simulink model "online_hardware_displacement_ctrl_arduino"  (R2020a)
settings: Solver=FixedStepAuto  StartTime=0.0  StopTime=25  FixedStep=0.01  RelTol=1e-3  EnableMultiTasking=on
libraries: simulink x4, arduinolib x4, arduinosensorlib x1
settings Model: SILPILModeSetting=veronly  ExtModeTrigDuration=2  Creator=Boreth  LastModifiedBy=Boreth
settings OptimizationCC: EnhancedBackFolding=on  PassReuseOutputArgsAs=Individual arguments  MaxStackSize=64  OptimizeBlockOrder=speed  DifferentSizesBufferReuse=on  EfficientTunableParamExpr=on
settings DebuggingCC: InheritedTsInSrcMsg=none  ParameterTunabilityLossMsg=error  ArithmeticOperatorsInVariantConditions=warning
settings HardwareCC: ProdBitPerPointer=32  ProdBitPerSizeT=32  ProdBitPerPtrDiffT=32  ProdLargestAtomicInteger=Long  ProdLargestAtomicFloat=Double  ProdWordSize=32  ProdHWDeviceType=ARM Compatible->ARM Cortex
settings SFSimCC: MATLABDynamicMemAlloc=off  CustomCodeUndefinedFunction=UseInterfaceOnly
settings RTWCC: SystemTargetFile=ert.tlc  HardwareBoard=Arduino Due  TLCOptions=-aInlineSetEventsForThisBaseRateFcn=TLC_FALSE -aSuppressMultiTaskScheduler=TLC_FALSE -aRateBasedStepFcn=1  TemplateMakefile=ert_default_tmf  GenerateReport=on  Toolchain=Arduino ARM  BuildConfiguration=Faster Runs  IncludeHyperlinkInReport=on  LaunchReport=on  GenerateTraceInfo=on  GenerateTraceReport=on  GenerateTraceReportSl=on  GenerateTraceReportSf=on  GenerateTraceReportEml=on
settings CodeAppCC: ForceParamTrailComments=on  IgnoreCustomStorageClasses=off  OperatorAnnotations=on  SimulinkDataObjDesc=on  SFDataObjDesc=on  InsertBlockDesc=on
settings ERTTargetCC: SupportContinuousTime=on  SupportVariableSizeSignals=on  ExtModeStaticAllocSize=24576

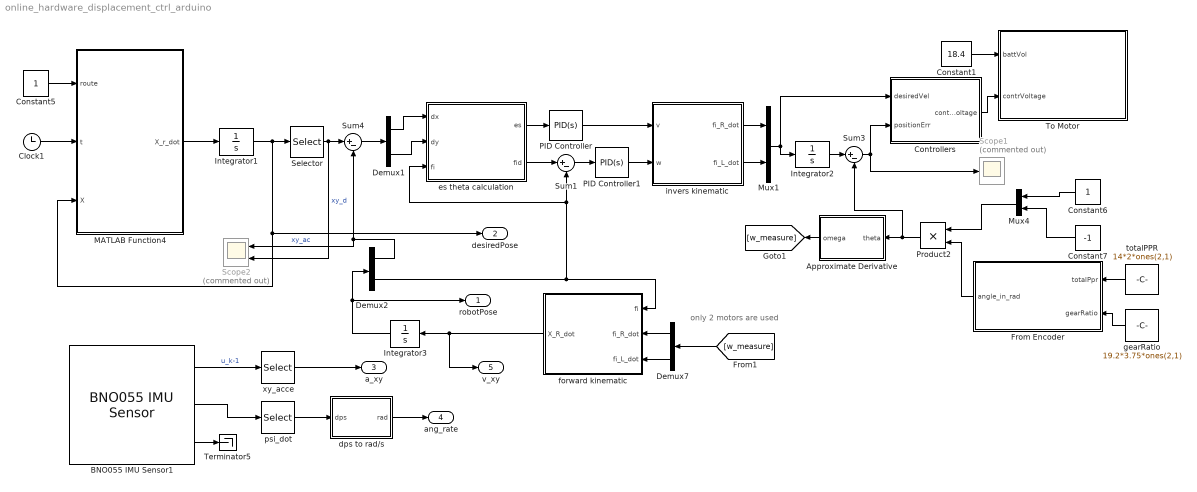
== system online_hardware_displacement_ctrl_arduino ==
  note: only 2 motors are used
  Approximate Derivative : Subsystem
  BNO055 IMU Sensor1 : arduinosensorlib/BNO055 IMU Sensor  SlaveAddress=0x28  OperationMode=Fusion  Accel=on  AngularRate=on  MagField=off  EulerAngles=off  Quat=off  LinearAccel=off  GravityVector=off  AccelRange=4G  AccelBW=62.5 Hz  GyroRange=2000 dps  GyroBW=32 Hz  MagODR=10 Hz  SampleTime=0.01  blockPlatform=ARDUINO
      settings: SourceProductName=Simulink Support Package for Arduino Hardware
  Clock1 : Clock
  Constant1 : Constant  Value=18.4
  Constant5 : Constant
  Constant6 : Constant
  Constant7 : Constant  Value=-1
  Controllers : Subsystem
  Demux1 : Demux  Outputs=2
  Demux2 : Demux  Outputs=[2 1]
  Demux7 : Demux  Outputs=2
  From Encoder : Subsystem
  Integrator1 : Integrator  InitialCondition=[0;0;0]
  Integrator2 : Integrator  InitialCondition=[0 0]
  Integrator3 : Integrator  InitialCondition=[0;0;0]
  MATLAB Function4 : MATLAB Function  TreatAsAtomicUnit=on
  Mux1 : Mux  Inputs=2
  Mux4 : Mux  Inputs=2
  PID Controller : simulink/Continuous/PID Controller  Controller=PID  Form=Parallel  TimeDomain=Continuous-time  UseExternalTs=off  SampleTime=-1  IntegratorMethod=Forward Euler  FilterMethod=Forward Euler  ControllerParametersSource=internal  P=0.35  I=0  D=0  UseFilter=on  N=100  TunerSelectOption=Transfer Function Based (PID Tuner App)  InitialConditionSource=internal  InitialConditionForIntegrator=0  InitialConditionForFilter=0  DifferentiatorICPrevScaledInput=0  ExternalReset=none  TrackingMode=off  Kt=1  LimitOutput=off  UpperSaturationLimit=inf  LowerSaturationLimit=-inf  LinearizeAsGain=on  AntiWindupMode=none  Kb=1  POutMin=[]  POutMax=[]  IOutMin=[]  IOutMax=[]  DOutMin=[]  DOutMax=[]  NOutMin=[]  NOutMax=[]  SumOutMin=[]  SumOutMax=[]  SaturationOutMin=[]  SaturationOutMax=[]  PParamMin=[]  PParamMax=[]  IParamMin=[]  IParamMax=[]  DParamMin=[]  DParamMax=[]  NParamMin=[]  NParamMax=[]  KbParamMin=[]  KbParamMax=[]  KtParamMin=[]  KtParamMax=[]  KbOutMin=[]  KbOutMax=[]  KtOutMin=[]  KtOutMax=[]  IntegratorOutMin=[]  IntegratorOutMax=[]  FilterOutMin=[]  FilterOutMax=[]  SumI1OutMin=[]  SumI1OutMax=[]  SumI2OutMin=[]  SumI2OutMax=[]  SumI3OutMin=[]  SumI3OutMax=[]  SumI4OutMin=[]  SumI4OutMax=[]  SumDOutMin=[]  SumDOutMax=[]  DifferentiatorOutMin=[]  DifferentiatorOutMax=[]  FilterDiffOutCoefMin=[]  FilterDiffOutCoefMax=[]  ReciprocalOutMin=[]  ReciprocalOutMax=[]  SumDenOutMin=[]  SumDenOutMax=[]  SumNumOutMin=[]  SumNumOutMax=[]  DivideOutMin=[]  DivideOutMax=[]  UdiffTsProdOutMin=[]  UdiffTsProdOutMax=[]  NTsProdOutMin=[]  NTsProdOutMax=[]  UintegralTsProdOutMin=[]  UintegralTsProdOutMax=[]  UngainTsProdOutMin=[]  UngainTsProdOutMax=[]  IntegratorContinuousStateAttributes=''  IntegratorStateMustResolveToSignalObject=off  IntegratorRTWStateStorageClass=Auto  FilterContinuousStateAttributes=''  FilterStateMustResolveToSignalObject=off  FilterRTWStateStorageClass=Auto  ParallelPVariant=InternalParameters  IdealPVariant=Disabled  IVariant=InternalParameters  DVariant=InternalParameters  IntegratorVariant=Continuous  SatVariant=Disabled  AWVariant=Passthrough  PCopyVariant=Disabled  TRVariant=Disabled  FdbkBlocksVariant=Forward  IdealPFdbkVariant=Disabled  SatFdbkVariant=Disabled  DerivativeFilterVariant=ContFilter  NVariant=InternalParameters  NCopyVariant=Disabled  FilterICVariant=InternalICsFilter  IntegratorICVariant=InternalICs  ExternalResetVariant=Disabled  TRSumVariant=Passthrough  SumFdbkVariant=Disabled  SumVariant=Sum_PID  TsampFilterVariant=InternalTs  TsampNgainVariant=Passthrough  TsampIntegralVariant=Passthrough
  PID Controller1 : simulink/Continuous/PID Controller  Controller=PID  Form=Parallel  TimeDomain=Continuous-time  UseExternalTs=off  SampleTime=-1  IntegratorMethod=Forward Euler  FilterMethod=Forward Euler  ControllerParametersSource=internal  P=3.2  I=0  D=0  UseFilter=on  N=100  TunerSelectOption=Transfer Function Based (PID Tuner App)  InitialConditionSource=internal  InitialConditionForIntegrator=0  InitialConditionForFilter=0  DifferentiatorICPrevScaledInput=0  ExternalReset=none  TrackingMode=off  Kt=1  LimitOutput=off  UpperSaturationLimit=inf  LowerSaturationLimit=-inf  LinearizeAsGain=on  AntiWindupMode=none  Kb=1  POutMin=[]  POutMax=[]  IOutMin=[]  IOutMax=[]  DOutMin=[]  DOutMax=[]  NOutMin=[]  NOutMax=[]  SumOutMin=[]  SumOutMax=[]  SaturationOutMin=[]  SaturationOutMax=[]  PParamMin=[]  PParamMax=[]  IParamMin=[]  IParamMax=[]  DParamMin=[]  DParamMax=[]  NParamMin=[]  NParamMax=[]  KbParamMin=[]  KbParamMax=[]  KtParamMin=[]  KtParamMax=[]  KbOutMin=[]  KbOutMax=[]  KtOutMin=[]  KtOutMax=[]  IntegratorOutMin=[]  IntegratorOutMax=[]  FilterOutMin=[]  FilterOutMax=[]  SumI1OutMin=[]  SumI1OutMax=[]  SumI2OutMin=[]  SumI2OutMax=[]  SumI3OutMin=[]  SumI3OutMax=[]  SumI4OutMin=[]  SumI4OutMax=[]  SumDOutMin=[]  SumDOutMax=[]  DifferentiatorOutMin=[]  DifferentiatorOutMax=[]  FilterDiffOutCoefMin=[]  FilterDiffOutCoefMax=[]  ReciprocalOutMin=[]  ReciprocalOutMax=[]  SumDenOutMin=[]  SumDenOutMax=[]  SumNumOutMin=[]  SumNumOutMax=[]  DivideOutMin=[]  DivideOutMax=[]  UdiffTsProdOutMin=[]  UdiffTsProdOutMax=[]  NTsProdOutMin=[]  NTsProdOutMax=[]  UintegralTsProdOutMin=[]  UintegralTsProdOutMax=[]  UngainTsProdOutMin=[]  UngainTsProdOutMax=[]  IntegratorContinuousStateAttributes=''  IntegratorStateMustResolveToSignalObject=off  IntegratorRTWStateStorageClass=Auto  FilterContinuousStateAttributes=''  FilterStateMustResolveToSignalObject=off  FilterRTWStateStorageClass=Auto  ParallelPVariant=InternalParameters  IdealPVariant=Disabled  IVariant=InternalParameters  DVariant=InternalParameters  IntegratorVariant=Continuous  SatVariant=Disabled  AWVariant=Passthrough  PCopyVariant=Disabled  TRVariant=Disabled  FdbkBlocksVariant=Forward  IdealPFdbkVariant=Disabled  SatFdbkVariant=Disabled  DerivativeFilterVariant=ContFilter  NVariant=InternalParameters  NCopyVariant=Disabled  FilterICVariant=InternalICsFilter  IntegratorICVariant=InternalICs  ExternalResetVariant=Disabled  TRSumVariant=Passthrough  SumFdbkVariant=Disabled  SumVariant=Sum_PID  TsampFilterVariant=InternalTs  TsampNgainVariant=Passthrough  TsampIntegralVariant=Passthrough
  Product2 : Product
  Scope1 : Scope  Commented=on
  Scope2 : Scope  Commented=on  NumInputPorts=2
  Selector : Selector  InputPortWidth=3  IndexOptions=Index vector (dialog)  Indices=[1 2]  OutputSizes=1
  Sum1 : Sum  Inputs=|+-
  Sum3 : Sum  Inputs=|+-
  Sum4 : Sum  Inputs=|+-
  Terminator5 : Terminator
  To Motor : Subsystem
  dps to rad/s : MATLAB Function  TreatAsAtomicUnit=on
  es theta calculation : MATLAB Function  TreatAsAtomicUnit=on
  forward kinematic : MATLAB Function  TreatAsAtomicUnit=on
  gearRatio : Constant  Value=19.2*3.75*ones(2,1)
  invers kinematic : MATLAB Function  TreatAsAtomicUnit=on
  psi_dot : Selector  InputPortWidth=3  IndexOptions=Index vector (dialog)  Indices=3  OutputSizes=1
  totalPPR : Constant  Value=14*2*ones(2,1)
  xy_acce : Selector  InputPortWidth=3  IndexOptions=Index vector (dialog)  Indices=[1 2]  OutputSizes=1
  robotPose : Outport
  desiredPose : Outport  Port=2
  a_xy : Outport  Port=3
  ang_rate : Outport  Port=4
  v_xy : Outport  Port=5
  wires:
  Approximate Derivative/1(omega) -> [w_measure]
  Controllers/1(contrVoltage) -> To Motor/2(contrVoltage)
  Mux1/1 -> Controllers/1(desiredVel), Integrator2/1
  Integrator2/1 -> Sum3/1
  From Encoder/1(angle_in_rad) -> Product2/2
  Sum3/1 -> Scope1/1, Controllers/2(positionErr)
  Mux4/1 -> Product2/1
  Product2/1 -> Sum3/2, Approximate Derivative/1(theta)
  Constant7/1 -> Mux4/2
  Constant6/1 -> Mux4/1
  BNO055 IMU Sensor1/3 -> Terminator5/1
  xy_acce/1 -> a_xy/1
  dps to rad/s/1(rad) -> ang_rate/1
  BNO055 IMU Sensor1/1 -> xy_acce/1  "u_k-1"
  psi_dot/1 -> dps to rad/s/1(dps)
  BNO055 IMU Sensor1/2 -> psi_dot/1
  forward kinematic/1(X_R_dot) -> v_xy/1, Integrator3/1
  Selector/1 -> Scope2/2, Sum4/1  "xy_d"
  PID Controller1/1 -> invers kinematic/2(w)
  Demux1/1 -> es theta calculation/1(dx)
  Demux1/2 -> es theta calculation/2(dy)
  MATLAB Function4/1(X_r_dot) -> Integrator1/1
  es theta calculation/2(fid) -> Sum1/1
  PID Controller/1 -> invers kinematic/1(v)
  Sum4/1 -> Demux1/1
  Demux2/2 -> es theta calculation/3(fi), Sum1/2, forward kinematic/1(fi)
  Sum1/1 -> PID Controller1/1
  es theta calculation/1(es) -> PID Controller/1
  Demux7/1 -> forward kinematic/2(fi_R_dot)
  Demux2/1 -> Scope2/1, Sum4/2  "xy_ac"
  invers kinematic/1(fi_R_dot) -> Mux1/1
  Demux7/2 -> forward kinematic/3(fi_L_dot)
  Integrator3/1 -> Demux2/1, robotPose/1
  invers kinematic/2(fi_L_dot) -> Mux1/2
  Clock1/1 -> MATLAB Function4/2(t)
  Integrator1/1 -> Selector/1, desiredPose/1, MATLAB Function4/3(X)
  Constant5/1 -> MATLAB Function4/1(route)
  [w_measure] -> Demux7/1
  totalPPR/1 -> From Encoder/1(totalPpr)
  gearRatio/1 -> From Encoder/2(gearRatio)
  Constant1/1 -> To Motor/1(battVol)

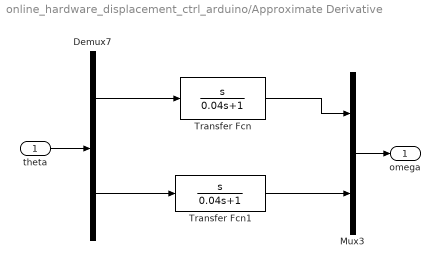
== system online_hardware_displacement_ctrl_arduino/Approximate Derivative ==
  theta : Inport
  Demux7 : Demux  Outputs=2
  Mux3 : Mux  Inputs=2
  Transfer Fcn : TransferFcn  Numerator=[1 0]  Denominator=[0.04 1]
  Transfer Fcn1 : TransferFcn  Numerator=[1 0]  Denominator=[0.04 1]
  omega : Outport
  wires:
  Transfer Fcn1/1 -> Mux3/2
  Transfer Fcn/1 -> Mux3/1
  Mux3/1 -> omega/1
  Demux7/1 -> Transfer Fcn/1
  Demux7/2 -> Transfer Fcn1/1
  theta/1 -> Demux7/1

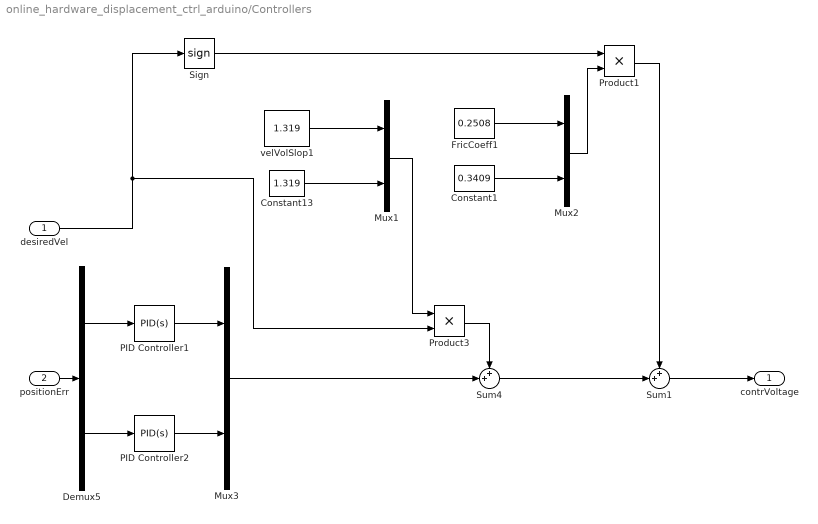
== system online_hardware_displacement_ctrl_arduino/Controllers ==
  desiredVel : Inport
  positionErr : Inport  Port=2
  Constant1 : Constant  Value=0.3409
  Constant13 : Constant  Value=1.319
  Demux5 : Demux  Outputs=2
  FricCoeff1 : Constant  Value=0.2508
  Mux1 : Mux  Inputs=2
  Mux2 : Mux  Inputs=2
  Mux3 : Mux  Inputs=2
  "PID Controller1 " : simulink/Continuous/PID Controller  Controller=PID  Form=Parallel  TimeDomain=Continuous-time  UseExternalTs=off  SampleTime=-1  IntegratorMethod=Forward Euler  FilterMethod=Forward Euler  ControllerParametersSource=internal  P=60  I=0  D=3  UseFilter=on  N=50  TunerSelectOption=Transfer Function Based (PID Tuner App)  InitialConditionSource=internal  InitialConditionForIntegrator=0  InitialConditionForFilter=0  DifferentiatorICPrevScaledInput=0  ExternalReset=none  TrackingMode=off  Kt=1  LimitOutput=off  UpperSaturationLimit=inf  LowerSaturationLimit=-inf  LinearizeAsGain=on  AntiWindupMode=none  Kb=1  POutMin=[]  POutMax=[]  IOutMin=[]  IOutMax=[]  DOutMin=[]  DOutMax=[]  NOutMin=[]  NOutMax=[]  SumOutMin=[]  SumOutMax=[]  SaturationOutMin=[]  SaturationOutMax=[]  PParamMin=[]  PParamMax=[]  IParamMin=[]  IParamMax=[]  DParamMin=[]  DParamMax=[]  NParamMin=[]  NParamMax=[]  KbParamMin=[]  KbParamMax=[]  KtParamMin=[]  KtParamMax=[]  KbOutMin=[]  KbOutMax=[]  KtOutMin=[]  KtOutMax=[]  IntegratorOutMin=[]  IntegratorOutMax=[]  FilterOutMin=[]  FilterOutMax=[]  SumI1OutMin=[]  SumI1OutMax=[]  SumI2OutMin=[]  SumI2OutMax=[]  SumI3OutMin=[]  SumI3OutMax=[]  SumI4OutMin=[]  SumI4OutMax=[]  SumDOutMin=[]  SumDOutMax=[]  DifferentiatorOutMin=[]  DifferentiatorOutMax=[]  FilterDiffOutCoefMin=[]  FilterDiffOutCoefMax=[]  ReciprocalOutMin=[]  ReciprocalOutMax=[]  SumDenOutMin=[]  SumDenOutMax=[]  SumNumOutMin=[]  SumNumOutMax=[]  DivideOutMin=[]  DivideOutMax=[]  UdiffTsProdOutMin=[]  UdiffTsProdOutMax=[]  NTsProdOutMin=[]  NTsProdOutMax=[]  UintegralTsProdOutMin=[]  UintegralTsProdOutMax=[]  UngainTsProdOutMin=[]  UngainTsProdOutMax=[]  IntegratorContinuousStateAttributes=''  IntegratorStateMustResolveToSignalObject=off  IntegratorRTWStateStorageClass=Auto  FilterContinuousStateAttributes=''  FilterStateMustResolveToSignalObject=off  FilterRTWStateStorageClass=Auto  ParallelPVariant=InternalParameters  IdealPVariant=Disabled  IVariant=InternalParameters  DVariant=InternalParameters  IntegratorVariant=Continuous  SatVariant=Disabled  AWVariant=Passthrough  PCopyVariant=Disabled  TRVariant=Disabled  FdbkBlocksVariant=Forward  IdealPFdbkVariant=Disabled  SatFdbkVariant=Disabled  DerivativeFilterVariant=ContFilter  NVariant=InternalParameters  NCopyVariant=Disabled  FilterICVariant=InternalICsFilter  IntegratorICVariant=InternalICs  ExternalResetVariant=Disabled  TRSumVariant=Passthrough  SumFdbkVariant=Disabled  SumVariant=Sum_PID  TsampFilterVariant=InternalTs  TsampNgainVariant=Passthrough  TsampIntegralVariant=Passthrough
  PID Controller2 : simulink/Continuous/PID Controller  Controller=PID  Form=Parallel  TimeDomain=Continuous-time  UseExternalTs=off  SampleTime=-1  IntegratorMethod=Forward Euler  FilterMethod=Forward Euler  ControllerParametersSource=internal  P=60  I=0  D=3  UseFilter=on  N=100  TunerSelectOption=Transfer Function Based (PID Tuner App)  InitialConditionSource=internal  InitialConditionForIntegrator=0  InitialConditionForFilter=0  DifferentiatorICPrevScaledInput=0  ExternalReset=none  TrackingMode=off  Kt=1  LimitOutput=off  UpperSaturationLimit=inf  LowerSaturationLimit=-inf  LinearizeAsGain=on  AntiWindupMode=none  Kb=1  POutMin=[]  POutMax=[]  IOutMin=[]  IOutMax=[]  DOutMin=[]  DOutMax=[]  NOutMin=[]  NOutMax=[]  SumOutMin=[]  SumOutMax=[]  SaturationOutMin=[]  SaturationOutMax=[]  PParamMin=[]  PParamMax=[]  IParamMin=[]  IParamMax=[]  DParamMin=[]  DParamMax=[]  NParamMin=[]  NParamMax=[]  KbParamMin=[]  KbParamMax=[]  KtParamMin=[]  KtParamMax=[]  KbOutMin=[]  KbOutMax=[]  KtOutMin=[]  KtOutMax=[]  IntegratorOutMin=[]  IntegratorOutMax=[]  FilterOutMin=[]  FilterOutMax=[]  SumI1OutMin=[]  SumI1OutMax=[]  SumI2OutMin=[]  SumI2OutMax=[]  SumI3OutMin=[]  SumI3OutMax=[]  SumI4OutMin=[]  SumI4OutMax=[]  SumDOutMin=[]  SumDOutMax=[]  DifferentiatorOutMin=[]  DifferentiatorOutMax=[]  FilterDiffOutCoefMin=[]  FilterDiffOutCoefMax=[]  ReciprocalOutMin=[]  ReciprocalOutMax=[]  SumDenOutMin=[]  SumDenOutMax=[]  SumNumOutMin=[]  SumNumOutMax=[]  DivideOutMin=[]  DivideOutMax=[]  UdiffTsProdOutMin=[]  UdiffTsProdOutMax=[]  NTsProdOutMin=[]  NTsProdOutMax=[]  UintegralTsProdOutMin=[]  UintegralTsProdOutMax=[]  UngainTsProdOutMin=[]  UngainTsProdOutMax=[]  IntegratorContinuousStateAttributes=''  IntegratorStateMustResolveToSignalObject=off  IntegratorRTWStateStorageClass=Auto  FilterContinuousStateAttributes=''  FilterStateMustResolveToSignalObject=off  FilterRTWStateStorageClass=Auto  ParallelPVariant=InternalParameters  IdealPVariant=Disabled  IVariant=InternalParameters  DVariant=InternalParameters  IntegratorVariant=Continuous  SatVariant=Disabled  AWVariant=Passthrough  PCopyVariant=Disabled  TRVariant=Disabled  FdbkBlocksVariant=Forward  IdealPFdbkVariant=Disabled  SatFdbkVariant=Disabled  DerivativeFilterVariant=ContFilter  NVariant=InternalParameters  NCopyVariant=Disabled  FilterICVariant=InternalICsFilter  IntegratorICVariant=InternalICs  ExternalResetVariant=Disabled  TRSumVariant=Passthrough  SumFdbkVariant=Disabled  SumVariant=Sum_PID  TsampFilterVariant=InternalTs  TsampNgainVariant=Passthrough  TsampIntegralVariant=Passthrough
  Product1 : Product
  Product3 : Product
  Sign : Signum
  Sum1 : Sum  Inputs=++|
  Sum4 : Sum  Inputs=++|
  velVolSlop1 : Constant  Value=1.319
  contrVoltage : Outport
  wires:
  PID Controller2/1 -> Mux3/2
  Demux5/1 -> "PID Controller1 "/1
  "PID Controller1 "/1 -> Mux3/1
  positionErr/1 -> Demux5/1
  Demux5/2 -> PID Controller2/1
  Constant13/1 -> Mux1/2
  velVolSlop1/1 -> Mux1/1
  Mux1/1 -> Product3/1
  Sum1/1 -> contrVoltage/1
  Mux3/1 -> Sum4/2
  desiredVel/1 -> Sign/1, Product3/2
  Sum4/1 -> Sum1/2
  FricCoeff1/1 -> Mux2/1
  Constant1/1 -> Mux2/2
  Sign/1 -> Product1/1
  Mux2/1 -> Product1/2
  Product1/1 -> Sum1/1
  Product3/1 -> Sum4/1

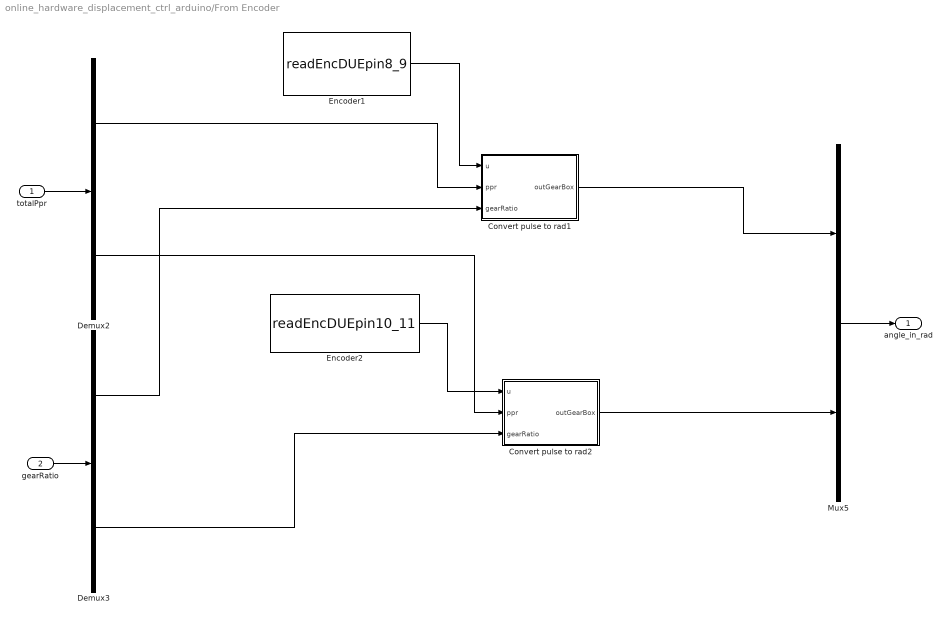
== system online_hardware_displacement_ctrl_arduino/From Encoder ==
  totalPpr : Inport
  gearRatio : Inport  Port=2
  Convert pulse to rad1 : MATLAB Function  TreatAsAtomicUnit=on
  Convert pulse to rad2 : MATLAB Function  TreatAsAtomicUnit=on
  Demux2 : Demux  Outputs=2
  Demux3 : Demux  Outputs=2
  Encoder1 : S-Function  InitFcn=try, set_param(gcb,'FunctionName','readEncDUEpin8_9'), end  FunctionName=readEncDUEpin8_9  SFunctionModules=readEncDUEpin8_9_wrapper  SFunctionDeploymentMode=off  EnableBusSupport=off  mask(S-Function Builder){}
      mask help: Simulink:masks:SFunctionBuilder_MD
      mask init:
      | val = [[.9  0.75 0.75 1 1 .9 .9 1]',[1 1 0.75 0.75 .9 .9 1 .9]'];try , sys = get_param(gcb,'SfunBuilderFcnName');if isempty(sys), sys = get_param(gcb,'FunctionName'); end,catch, sys = get_param(gcb,'FunctionName'); end
      settings: CopyFcn=set_param(gcbh,'LinkStatus','none')  PreSaveFcn=try, set_param(gcb,'FunctionName','readEncDUEpin8_9'), end  OpenFcn=sfunctionwizard(gcbh)
      mask Display: plot(val(:,1),val(:,2)),disp(sys), port_label('output',1,'count')
  Encoder2 : S-Function  InitFcn=try, set_param(gcb,'FunctionName','readEncDUEpin10_11'), end  FunctionName=readEncDUEpin10_11  SFunctionModules=readEncDUEpin10_11_wrapper  SFunctionDeploymentMode=off  EnableBusSupport=off  mask(S-Function Builder){}
      mask help: Simulink:masks:SFunctionBuilder_MD
      mask init: same as online_hardware_displacement_ctrl_arduino/From Encoder/Encoder1
      settings: CopyFcn=set_param(gcbh,'LinkStatus','none')  PreSaveFcn=try, set_param(gcb,'FunctionName','readEncDUEpin10_11'), end  OpenFcn=sfunctionwizard(gcbh)
      mask Display: plot(val(:,1),val(:,2)),disp(sys), port_label('output',1,'countt')
  Mux5 : Mux  Inputs=2
  angle_in_rad : Outport
  wires:
  Demux3/1 -> Convert pulse to rad1/3(gearRatio)
  Mux5/1 -> angle_in_rad/1
  Demux2/2 -> Convert pulse to rad2/2(ppr)
  gearRatio/1 -> Demux3/1
  Encoder2/1 -> Convert pulse to rad2/1(u)
  Demux2/1 -> Convert pulse to rad1/2(ppr)
  Convert pulse to rad1/1(outGearBox) -> Mux5/1
  Demux3/2 -> Convert pulse to rad2/3(gearRatio)
  Convert pulse to rad2/1(outGearBox) -> Mux5/2
  totalPpr/1 -> Demux2/1
  Encoder1/1 -> Convert pulse to rad1/1(u)

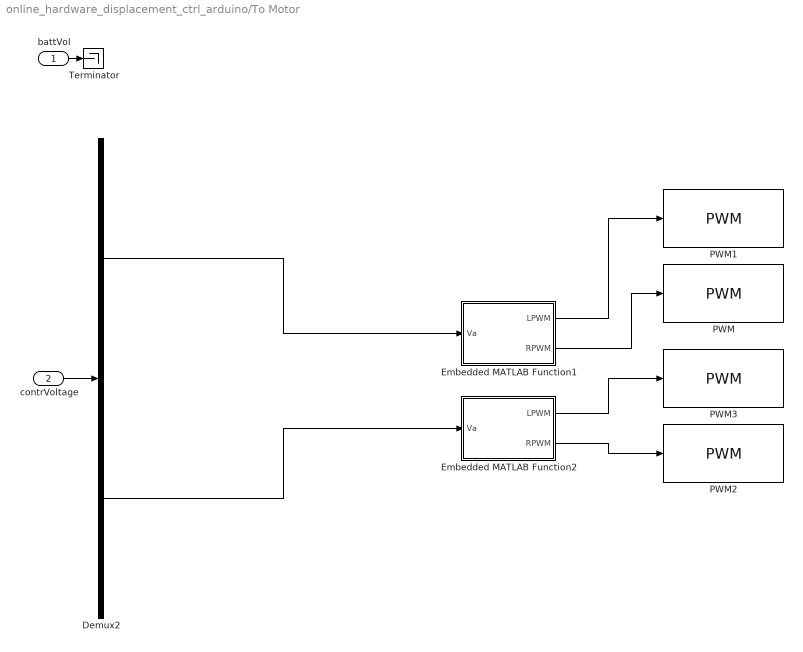
== system online_hardware_displacement_ctrl_arduino/To Motor ==
  battVol : Inport
  contrVoltage : Inport  Port=2
  Demux2 : Demux  Outputs=2
  Embedded MATLAB Function1 : MATLAB Function  TreatAsAtomicUnit=on
  Embedded MATLAB Function2 : MATLAB Function  TreatAsAtomicUnit=on
  PWM : arduinolib/PWM  pinNumber=6  frequencyType=Default  desiredFrequency=490.2  achievableFrequency=490.2
  PWM1 : arduinolib/PWM  pinNumber=7  frequencyType=Default  desiredFrequency=490.2  achievableFrequency=490.2
  PWM2 : arduinolib/PWM  pinNumber=4  frequencyType=Default  desiredFrequency=490.2  achievableFrequency=490.2
  PWM3 : arduinolib/PWM  pinNumber=5  frequencyType=Default  desiredFrequency=490.2  achievableFrequency=490.2
  Terminator : Terminator
  wires:
  contrVoltage/1 -> Demux2/1
  Embedded MATLAB Function1/1(LPWM) -> PWM1/1
  Embedded MATLAB Function1/2(RPWM) -> PWM/1
  Embedded MATLAB Function2/1(LPWM) -> PWM3/1
  Embedded MATLAB Function2/2(RPWM) -> PWM2/1
  battVol/1 -> Terminator/1
  Demux2/1 -> Embedded MATLAB Function1/1(Va)
  Demux2/2 -> Embedded MATLAB Function2/1(Va)

== matlab function online_hardware_displacement_ctrl_arduino/MATLAB Function4 ==
  settings: updateMethod=DISCRETE
  data: route input; t input; X_r_dot output; X input
function X_r_dot = fcn(route,t,X)
%#codegen

persistent k i j X_p_i omega_p_j t1 t2
if isempty(k)
    i = int8(1);
    j = int8(1);
    X_p_i = [0;0];
    omega_p_j = 0;
    t1 = t;
    t2 = t;
    k = 1;
end
tau = 0.15;
tau1 = 0.15;
V_max = 0.5; % maximum velocity
a = 0.5;      % acceleration
omega_max = 0.5;
alpha = 50.3;

X_r_dot = zeros(3,1);
switch route
    case 1
%         X_p = [1.5   1.5  0];
        X_p = [3   0  0
               3    3   0
               0    3   0
               0    0   0
               ]; % X_p = [x,y,theta];
    otherwise
        X_r_dot = [0;0;0];
        return;
end
X_p = X_p'; % X_p = [x;y;theta]
[~,col] = size(X_p);
dX = X_p(1:2,i)-X_p_i;
norm_dX = norm(dX);
two_rmin = V_max^2/a;
dtheta = X_p(3,j)-omega_p_j;
norm_dtheta = abs(dtheta);
two_thetamin = omega_max^2/alpha;

if norm_dX > two_rmin
    ta = V_max/a;                   % acceleration period
    tad = (norm_dX-two_rmin)/V_max; % acc to deceleration period
    td = ta + tad;                  % start deceleration
    te = ta + td;                   % end deceleration
    if (t-t1) < ta
        v = a*(t-t1);
    elseif ta <= (t-t1) && (t-t1) < td
        v = V_max;
    elseif td <= (t-t1) && (t-t1) < te
        v = -a*(t-t1-td) + V_max;
    else
        v = 0;
    end
else
    tp = sqrt(norm_dX/a);
    te = 2*tp;
    Vp = a*tp;
    if (t-t1) < tp
        v = a*(t-t1);
    elseif tp < (t-t1) && (t-t1) < te
        v = -a*(t-t1-tp)+Vp;
    else
        v = 0;
    end
end
if norm_dX~=0
    X_r_dot(1:2) = v*dX/norm_dX;
end

dist_X = norm(X_p(1:2,i)-X(1:2));
if (i<col)&&(dist_X < tau)
    X_p_i = X(1:2);
    t1    = t;
    i     = i+1;
end

if norm_dtheta > two_thetamin
    ta = omega_max/alpha;                   % acceleration period
    tad = (norm_dtheta-two_thetamin)/omega_max; % acc to deceleration period
    td = ta + tad;                  % start deceleration
    te = ta + td;                   % end deceleration
    if (t-t2) < ta
        omega = alpha*(t-t2);
    elseif ta <= (t-t2) && (t-t2) < td
        omega = omega_max;
    elseif td <= (t-t2) && (t-t2) < te
        omega = -alpha*(t-t2-td) + omega_max;
    else
        omega = 0;
    end
else
    tp = sqrt(norm_dtheta/alpha);
    te = 2*tp;
    omegap = alpha*tp;
    if (t-t2) < tp
        omega = alpha*(t-t2);
    elseif tp < (t-t2) && (t-t2) < te
        omega = -alpha*(t-t2-tp)+omegap;
    else
        omega = 0;
    end
end
X_r_dot(3) = omega*sign(dtheta);

dist_theta = abs(X_p(3,j)-X(3));
if (j<col)&&(dist_theta < tau1)
    omega_p_j = X(3);
    t2    = t;
    j     = j+1;
end

== matlab function online_hardware_displacement_ctrl_arduino/From Encoder/Convert pulse to rad1 ==
  settings: updateMethod=DISCRETE
  data: u input; ppr input; gearRatio input; outGearBox output
function outGearBox = fcn(u,ppr,gearRatio)

persistent counter_num over_flag
if(isempty(counter_num)), counter_num = 0;end
if(isempty(over_flag)), over_flag = 0;end
pulse2radian = 2*pi/ppr; % 1 pulse = ?? radian

if(double(u) - counter_num > 40000), over_flag = over_flag-1;
elseif(double(u) - counter_num < -40000), over_flag = over_flag+1;
end

inGearBox = (double(u)+over_flag*(2^32 -1))*pulse2radian; 
outGearBox = inGearBox/gearRatio;
counter_num = double(u) ;

== matlab function online_hardware_displacement_ctrl_arduino/From Encoder/Convert pulse to rad2 ==
  settings: updateMethod=DISCRETE
  data: u input; ppr input; gearRatio input; outGearBox output
function outGearBox = fcn(u,ppr,gearRatio)

persistent counter_num over_flag
if(isempty(counter_num)), counter_num = 0;end
if(isempty(over_flag)), over_flag = 0;end
pulse2radian = 2*pi/ppr; % 1 pulse = ?? radian

if(double(u) - counter_num > 40000), over_flag = over_flag-1;
elseif(double(u) - counter_num < -40000), over_flag = over_flag+1;
end

inGearBox = (double(u)+over_flag*(2^32 -1))*pulse2radian; 
outGearBox = inGearBox/gearRatio;
counter_num = double(u) ;

== matlab function online_hardware_displacement_ctrl_arduino/es theta calculation ==
  data: es output; dx input; fid output; dy input; fi input
function [es, fid]   = fcn(dx, dy, fi)
% es & theta calculation
fid = atan2(dy,dx);
es = sqrt(dy^2 + dx^2)*cos(fid - fi);

== matlab function online_hardware_displacement_ctrl_arduino/To Motor/Embedded MATLAB Function1 ==
  data: Va input; LPWM output; RPWM output
function [LPWM,RPWM] = fcn(Va)

Vmax = 18.4; % supply voltage is Vmax = 18.4v
PWM = abs(Va)*255/Vmax;
if PWM > 255
    PWM = 255;
end
if Va>=0
    LPWM = PWM;
    RPWM = 0;
else
    LPWM = 0;
    RPWM = PWM;
end

== matlab function online_hardware_displacement_ctrl_arduino/dps to rad//s ==
  data: dps input; rad output
function rad = fcn(dps)

rad = dps*pi/180;

== matlab function online_hardware_displacement_ctrl_arduino/To Motor/Embedded MATLAB Function2 ==
  data: Va input; LPWM output; RPWM output
function [LPWM,RPWM] = fcn(Va)

Vmax = 18.4; % supply voltage is Vmax = 18.4v
PWM = abs(Va)*255/Vmax;
if PWM > 255
    PWM = 255;
end
if Va>=0
    LPWM = PWM;
    RPWM = 0;
else
    LPWM = 0;
    RPWM = PWM;
end

== matlab function online_hardware_displacement_ctrl_arduino/forward kinematic ==
  data: fi input; fi_R_dot input; X_R_dot output; fi_L_dot input
function X_R_dot = B(fi,fi_R_dot, fi_L_dot)
%Forward Kinematic
r = 0.07;      %wheel radius
b = 0.22; 

v = r*[0.5 0.5]*[fi_R_dot; fi_L_dot];
w = r*[0.5/b -0.5/b]*[fi_R_dot; fi_L_dot];
X_R_dot = [cos(fi) 0;sin(fi) 0; 0 1]*[v; w];

== matlab function online_hardware_displacement_ctrl_arduino/invers kinematic ==
  data: v input; fi_R_dot output; w input; fi_L_dot output
function [fi_R_dot, fi_L_dot] = B_inv(v, w)
%Invers Kinematic
r = 0.07;      %wheel radius
b = 0.22; 
fi_R_dot = (v + w*b)/r;
fi_L_dot = (v - w*b)/r;
